simulink model "virt_model_stage_3"  (R2016a)
settings: Solver=VariableStepAuto  StartTime=0.0  StopTime=50  RelTol=1e-3
settings Model: Creator=maximilian  LastModifiedBy=maximilian

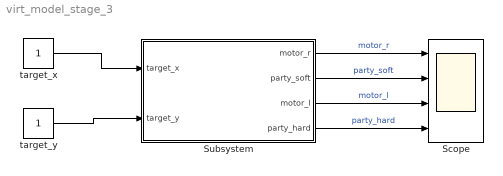
== system virt_model_stage_3 ==
  Scope : Scope  NumInputPorts=4
  Subsystem : Subsystem
  target_x : Constant
  target_y : Constant
  wires:
  target_x/1 -> Subsystem/1(target_x)
  target_y/1 -> Subsystem/2(target_y)
  Subsystem/1(motor_r) -> Scope/1  "motor_r"
  Subsystem/2(party_soft) -> Scope/2  "party_soft"
  Subsystem/3(motor_l) -> Scope/3  "motor_l"
  Subsystem/4(party_hard) -> Scope/4  "party_hard"

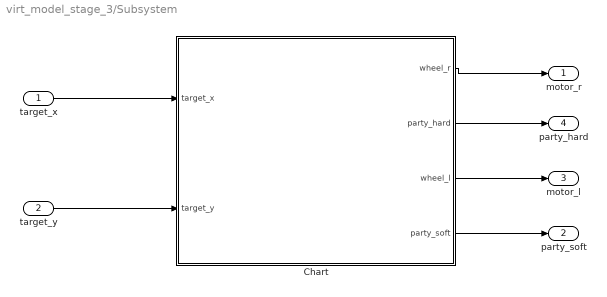
== system virt_model_stage_3/Subsystem ==
  target_x : Inport
  target_y : Inport  Port=2
  Chart : Stateflow chart  TreatAsAtomicUnit=on
  motor_r : Outport
  party_soft : Outport  Port=2
  motor_l : Outport  Port=3
  party_hard : Outport  Port=4
  wires:
  Chart/1(wheel_r) -> motor_r/1
  Chart/3(wheel_l) -> motor_l/1
  Chart/2(party_hard) -> party_hard/1
  target_x/1 -> Chart/1(target_x)
  target_y/1 -> Chart/2(target_y)
  Chart/4(party_soft) -> party_soft/1

== stateflow chart virt_model_stage_3/Subsystem/Chart ==
  state compute
    entry:
    target_dir = atan2((target_y - curr_y), (target_x - curr_x))
    dir = (target_dir - curr_dir) / rad_per_sec
    dist = sqrt((target_y - curr_y)^2 + (target_x - curr_x)^2) / dist_per_sec
  state rotate_left
    entry:
    wheel_r = 1
    wheel_l = -1
  state rotate_right
    entry:
    wheel_r = -1
    wheel_l = 1
  state drive
    entry:
    party_soft = 1
    wheel_r = 1
    wheel_l = 1
  state profit
    entry:
    party_hard = 1
    wheel_l = 0
    wheel_r = 0
  (default) -> compute : {curr_x = 0; curr_y = 0; curr_dir = 0}
  compute -> rotate_right [order 2] : [dir < 0]
  compute -> drive [order 3] : [dir == 0]
  compute -> rotate_left [order 1] : [dir > 0]
  rotate_right -> drive : [after(dir, sec)]
  rotate_left -> drive : [after(dir, sec)]
  drive -> profit : [after(dist, sec)]
  data: dist_per_sec constant double =0.1; target_x input; target_y input; rad_per_sec constant double =0.1; wheel_r output; party_hard output; wheel_l output; target_dir local; curr_y local; curr_x local; dir local; curr_dir local; dist local; party_soft output
